simulink model "drivecar"  (R2020b)
settings: Solver=VariableStepAuto  StartTime=0.0  StopTime=10.0  RelTol=1e-3
settings Model: Creator=Ege  LastModifiedBy=Ege

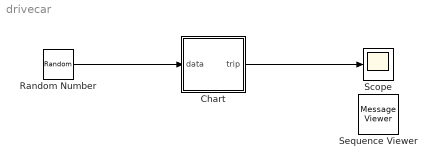
== system drivecar ==
  Chart : Stateflow chart  TreatAsAtomicUnit=on
  Random Number : RandomNumber  Mean=280  Variance=150  SampleTime=0.1
  Scope : Scope
  Sequence Viewer : MessageViewer  History=1000  SavedRootId=#
  wires:
  Random Number/1 -> Chart/1(data)
  Chart/1(trip) -> Scope/1

== stateflow chart drivecar/Chart ==
  state Driver [parallel]
    settings: executionOrder=1
    state Waiting_In_Parking
      ex:
      trip=data
    state Driving
      du:
      trip=trip-x
    state Reaching_Destination
      en:
      send(DestinationReached,Car)
    (default) -> Waiting_In_Parking
    Waiting_In_Parking -> Driving : [data>300]{send(SthHappened,Car)}
    Reaching_Destination -> Waiting_In_Parking : [x==0]
    Driving -> Driving [commented out] : after(1,sec)
    Driving -> Reaching_Destination : [trip<=0]
  state Car [parallel]
    settings: executionOrder=2
    state Idling
      en:
      x=0;
    state Deceleration
      en:
      x=x-1
    state Acceleration
      en:
      x=x+1
    state Cruising
    (default) -> Idling
    Idling -> Acceleration : SthHappened
    (junction 22) -> Idling [order 1] : [x<=0]
    (junction 22) -> Deceleration [order 2]
    (junction 24) -> Acceleration [order 2]
    Deceleration -> (junction 22) : after(1,sec)
    Cruising -> Deceleration : DestinationReached
    Acceleration -> (junction 24) : after(1,sec)
    (junction 24) -> Cruising [order 1] : [x>=10]
  data: data input; x local; trip output
  events: SthHappened local FUNCTION_CALL_EVENT; DestinationReached local FUNCTION_CALL_EVENT
